simulink model "Sim_Forcing_003h_expe_infra_transz_lim"  (Simulink 7.4)
settings: Solver=FixedStepDiscrete  StartTime=0.0  StopTime=inf  FixedStep=0.004  RelTol=1e-3
undefined symbols (not defined in the file or in its folder): DiscIntNeverNeededParam
libraries: simulink x39, gt_rt_lib x22, xpcutilitieslib x4, xpclib x2, dspswit3 x1
(part 1 of 4)
CloseFcn:
  | rtwprivate ssgencode ModelCloseRequest test
settings Model: Creator=traenkle  LastModifiedBy=iMose1  SimulationMode=external  ExtModeTrigDuration=10000
settings OptimizationCC: LocalBlockOutputs=off  InitFltsAndDblsToZero=on
settings DebuggingCC: AlgebraicLoopMsg=error  ArtificialAlgebraicLoopMsg=error  SaveWithParameterizedLinksMsg=none  BlockPriorityViolationMsg=error  MinStepSizeMsg=error
settings HardwareCC: TargetEndianess=LittleEndian  TargetHWDeviceType=MATLAB Host
settings RTWCC: SystemTargetFile=gt_rt.tlc  TemplateMakefile=gt_rt.tmf  Description=GIGATRONIK Real-Time Target  ProcessScript=gt_rt_make_rtw_hook
settings STFCustomTargetCC: ModelReferenceCompliant=off  GeneratePreprocessorConditionals=Disable all  MatFileLogging=on  SystemTargetFile=gt_rt.tlc
settings GRTTargetCC: ModelReferenceCompliant=off  ParMdlRefBuildCompliant=off  CompOptLevelCompliant=off  ExtMode=on  ExtModeMexArgs='192.168.102.111'
settings CustomProperty: DataType=string  Value=gtrt

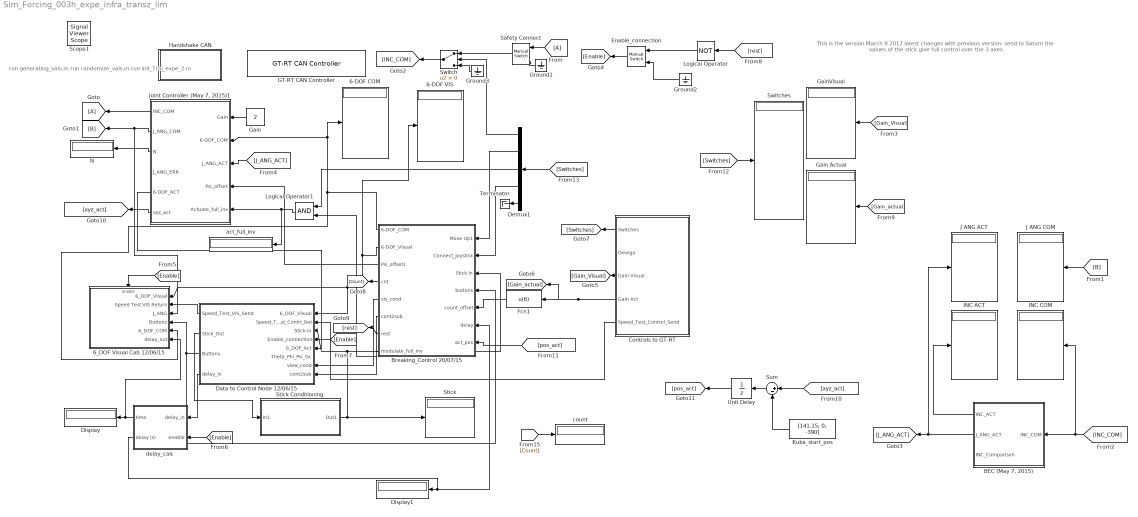
== system Sim_Forcing_003h_expe_infra_transz_lim ==
  note: This is the version
      | March 9 2017
      |
      | latest changes with previous version:
      | send to Saturn the values of the stick
      | give full control over the 3 axes
  note: run generating_vals.m
      | run randomize_vals.m
      | run init_Traj_expe_2.m
  6-DOF COM : Display
  6-DOF VIS : Display
  6_DOF Visual Cab 12/06/15 : Subsystem
  "BEC (May 7, 2015)" : Subsystem
  Breaking_Control 20/07/15 : Subsystem
  Controls to GT-RT : Subsystem
  Data to Control Node 12/06/15 : Subsystem
  Demux1 : Demux  Outputs=[1,1,1,3,4]
  Display : Display
  Display1 : Display
  Enable_connection : simulink/Signal Routing/Manual Switch  SystemSampleTime=-1  sw=1  action=0  varsize=off
  Fcn1 : Fcn  Expr=u(6)
  GT-RT CAN Controller : gt_rt_lib/GT-RT CAN Controller  uri='gt_rt_dev://localhost/dev/can0#0'  options='baudrate=500'
  Gain : Constant  Value=2  OutDataType=fixdt(1, 16)  OutScaling=2^0
  Gain Actual : Display
  GainVisual : Display
  Ground1 : Ground
  Ground2 : Ground
  Ground3 : Ground
  Handshake CAN : Subsystem
  INC ACT : Display
  INC COM : Display
  J ANG ACT : Display
  J ANG COM : Display
  "Joint Controller (May 7, 2015)1" : Subsystem
  Kuka_start_pos : Constant  Value=[141.15; 0; -390]  OutDataType=fixdt(1, 16)  OutScaling=2^0
  Logical Operator : Logic  Operator=NOT  AllPortsSameDT=off  OutDataTypeMode=boolean  LogicDataType=fixdt(0, 8)  OutDataTypeStr=boolean
  Logical Operator1 : Logic  AllPortsSameDT=off  OutDataTypeMode=boolean  LogicDataType=fixdt(0, 8)  OutDataTypeStr=boolean
  N : Display
  Safety Connect : simulink/Signal Routing/Manual Switch  SystemSampleTime=-1  sw=1  action=0  varsize=off
  Stick : Display
      settings: Decimation=40
  Stick Conditioning : Subsystem
  Sum : Sum  Inputs=|+-  OutDataType=fixdt(1, 16)  OutScaling=2^0
  Switch : Switch  Criteria=u2 > Threshold  OutDataType=fixdt(1, 16)  OutScaling=2^0
  Switches : Display
  Terminator : Terminator
  Unit Delay : UnitDelay  X0=[0 0 0]  SampleTime=-1
  act_full_inv : Display
  count : Display
      settings: Decimation=40
  delay_calc : Subsystem
  Scope1 : SignalViewerScope  IOType=viewer  ZoomMode=xonly  LegendLocations="524.3333           184           121      20.33333"  RefreshTime=0.035000
      settings: ShowLegends=on  TimeRange=10  YMin=2  YMax=3
  wires:
  Gain/1 -> "Joint Controller (May 7, 2015)1"/1(Gain)
  "Joint Controller (May 7, 2015)1"/1(INC_COM) -> [A]
  [A] -> Safety Connect/1
  "Joint Controller (May 7, 2015)1"/2(J_ANG_COM) -> [B], 6_DOF Visual Cab 12/06/15/3(J_ANG)
  "Joint Controller (May 7, 2015)1"/5(6-DOF_ACT) -> Data to Control Node 12/06/15/5(6_DOF_Act)
  [J_ANG_ACT] -> "Joint Controller (May 7, 2015)1"/3(J_ANG_ACT)
  "Joint Controller (May 7, 2015)1"/3(N) -> N/1
  Safety Connect/1 -> Switch/1
  Controls to GT-RT/3(Gain Visual) -> [Gain_Visual]
  Stick Conditioning/1(Out1) -> Stick/1, Breaking_Control 20/07/15/3(Stick In), Data to Control Node 12/06/15/3(Stick in)
  Data to Control Node 12/06/15/1(Speed_Test_VIS_Send) -> 6_DOF Visual Cab 12/06/15/2(Speed Test VIS Return)
  Controls to GT-RT/1(Switches) -> [Switches]
  Demux1/2 -> Breaking_Control 20/07/15/1(Move Up1)
  "BEC (May 7, 2015)"/2(J_ANG_ACT) -> [J_ANG_ACT], J ANG ACT/1
  Ground1/1 -> Safety Connect/2
  Ground3/1 -> Switch/3
  Demux1/1 -> Switch/2
  "BEC (May 7, 2015)"/1(INC_ACT) -> INC ACT/1
  [B] -> J ANG COM/1
  Switch/1 -> [INC_COM]
  [INC_COM] -> INC COM/1, "BEC (May 7, 2015)"/1(INC_COM)
  Breaking_Control 20/07/15/1(6-DOF_COM) -> 6-DOF COM/1, "Joint Controller (May 7, 2015)1"/2(6-DOF_COM), 6_DOF Visual Cab 12/06/15/5(6_DOF_COM)
  Demux1/4 -> Breaking_Control 20/07/15/2(Connect_Joystick)
  Demux1/5 -> Terminator/1
  Data to Control Node 12/06/15/3(Buttons) -> 6_DOF Visual Cab 12/06/15/4(Buttons), Breaking_Control 20/07/15/4(buttons)
  Breaking_Control 20/07/15/2(6-DOF_Visual) -> 6-DOF VIS/1, 6_DOF Visual Cab 12/06/15/1(6_DOF_Visual), Data to Control Node 12/06/15/1(6_DOF_Visual)
  Breaking_Control 20/07/15/3(Psi_offset1) -> "Joint Controller (May 7, 2015)1"/4(Psi_offset)
  Data to Control Node 12/06/15/4(delay_in) -> delay_calc/1(delay_in)
  delay_calc/1(time) -> Display/1, 6_DOF Visual Cab 12/06/15/6(delay_out)
  delay_calc/2(delay (s)) -> Display1/1, Breaking_Control 20/07/15/6(delay)
  Ground2/1 -> Enable_connection/2
  [Enable] -> 6_DOF Visual Cab 12/06/15/Enable
  [Enable] -> delay_calc/2(enable)
  [Enable] -> Data to Control Node 12/06/15/4(Enable_connection)
  [Gain_Visual] -> GainVisual/1
  [Gain_actual] -> Gain Actual/1
  Controls to GT-RT/4(Gain Act) -> [Gain_actual], Fcn1/1
  [Switches] -> Switches/1
  [Switches] -> Demux1/1
  Controls to GT-RT/5(Speed_Test_Control_Send) -> Data to Control Node 12/06/15/2(Speed_Test_Contrl_Ret)
  Enable_connection/1 -> [Enable]
  [Count] -> count/1
  Breaking_Control 20/07/15/4(cnt) -> [Count]
  Breaking_Control 20/07/15/5(vis_cond) -> Data to Control Node 12/06/15/7(view_cond)
  Breaking_Control 20/07/15/6(cont2sub) -> Data to Control Node 12/06/15/8(cont2sub)
  Breaking_Control 20/07/15/7(rest) -> [rest]
  [rest] -> Logical Operator/1
  Fcn1/1 -> Breaking_Control 20/07/15/5(count_offset)
  Unit Delay/1 -> [pos_act]
  [pos_act] -> Breaking_Control 20/07/15/7(act_pos)
  "Joint Controller (May 7, 2015)1"/6(xyz_act) -> [xyz_act]
  Sum/1 -> Unit Delay/1
  [xyz_act] -> Sum/1
  Kuka_start_pos/1 -> Sum/2
  Demux1/3 -> Logical Operator1/1
  Breaking_Control 20/07/15/8(modulate_full_inv) -> Logical Operator1/2
  Logical Operator1/1 -> "Joint Controller (May 7, 2015)1"/5(Actuate_full_inv), act_full_inv/1
  Logical Operator/1 -> Enable_connection/1
  Data to Control Node 12/06/15/2(Stick_Out) -> Stick Conditioning/1(In1)

== system Sim_Forcing_003h_expe_infra_transz_lim/6_DOF Visual Cab 12/06/15 ==
  note: send to visual node
  6_DOF_Visual : Inport
  Speed Test VIS Return : Inport  Port=2
  J_ANG : Inport  Port=3
  Buttons : Inport  Port=4
  6_DOF_COM : Inport  Port=5
  delay_out : Inport  Port=6
  Enable : EnablePort
  "Byte Packing " : xpcutilitieslib/Byte Packing   MaskPackedDataType=uint8  MaskUnpackedDataTypes={'single','single','single'}  MaskAlignment=1
  Constant2 : Constant  Value=9200  OutDataTypeMode=uint16  OutDataType=fixdt(1, 16)  OutScaling=2^0  OutDataTypeStr=uint16
  Constant3 : Constant  Value=32  OutDataTypeMode=uint32  OutDataType=fixdt(1, 16)  OutScaling=2^0  OutDataTypeStr=uint32
  Data Type Conversion : DataTypeConversion  OutDataTypeMode=single  OutDataType=fixdt(1, 16)  OutScaling=2^0  OutDataTypeStr=single
  Data Type Conversion1 : DataTypeConversion  OutDataTypeMode=single  OutDataType=fixdt(1, 16)  OutScaling=2^0  OutDataTypeStr=single
  Data Type Conversion6 : DataTypeConversion  OutDataTypeMode=single  OutDataType=fixdt(1, 16)  OutScaling=2^0  OutDataTypeStr=single
  GT-RT UDP  Write : gt_rt_lib/GT-RT UDP  Controller  uri='gtp://localhost/udp?port=9200'
  GT-RT UDP TX : gt_rt_lib/GT-RT UDP TX  uri='gtp://localhost/udp?port=9200'  hostname='192.168.102.13'
  Write Error : Display
  wires:
  Constant2/1 -> GT-RT UDP TX/2
  GT-RT UDP TX/1 -> Write Error/1
  Constant3/1 -> GT-RT UDP TX/4
  "Byte Packing "/1 -> GT-RT UDP TX/3
  Speed Test VIS Return/1 -> Data Type Conversion1/1
  6_DOF_Visual/1 -> Data Type Conversion/1
  Data Type Conversion1/1 -> "Byte Packing "/2
  Data Type Conversion/1 -> "Byte Packing "/1
  delay_out/1 -> Data Type Conversion6/1
  Data Type Conversion6/1 -> "Byte Packing "/3

== system Sim_Forcing_003h_expe_infra_transz_lim/BEC (May 7, 2015) ==
  INC_COM : Inport
  CAN Receive : Subsystem
  CAN Send : Subsystem
  Demux : Demux  Outputs=6
  Demux1 : Demux  Outputs=6
  Mux : Mux  Inputs=6
  Mux2 : Mux  Inputs=6
  Software limit switches : Subsystem
  Sum1 : Sum  Inputs=-+|  OutDataType=fixdt(1, 16)  OutScaling=2^0
  velocity and acceleration limitation : Subsystem
  INC_ACT : Outport
  J_ANG_ACT : Outport  Port=2
  INC_Comparison : Outport  Port=3
  wires:
  CAN Receive/7(New Data Flag (93)) -> CAN Send/1(New data flag (93))
  velocity and acceleration limitation/3(A3) -> Mux2/3
  velocity and acceleration limitation/6(A6) -> Mux2/6
  velocity and acceleration limitation/1(A1) -> Mux2/1
  velocity and acceleration limitation/2(A2) -> Mux2/2
  velocity and acceleration limitation/4(A4) -> Mux2/4
  velocity and acceleration limitation/5(A5) -> Mux2/5
  Software limit switches/1(Out1) -> velocity and acceleration limitation/1(In1)
  Software limit switches/2(Out2) -> velocity and acceleration limitation/2(In2)
  Software limit switches/3(Out3) -> velocity and acceleration limitation/3(In3)
  Software limit switches/4(Out4) -> velocity and acceleration limitation/4(In4)
  Software limit switches/5(Out5) -> velocity and acceleration limitation/5(In5)
  Software limit switches/6(Out6) -> velocity and acceleration limitation/6(In6)
  CAN Receive/1(Act_Axis1 [deg]) -> Mux/1
  CAN Receive/2(Act_Axis2  [deg]) -> Mux/2
  CAN Receive/3(Act_Axis3  [deg]) -> Mux/3
  CAN Receive/4(Act_Axis4 [deg]) -> Mux/4
  CAN Receive/5(Act_Axis5 [deg]) -> Mux/5
  CAN Receive/6(Act_Axis6 [deg]) -> Mux/6
  Demux/1 -> Software limit switches/1(In1)
  Demux/2 -> Software limit switches/2(In2)
  Demux/3 -> Software limit switches/3(In3)
  Demux/4 -> Software limit switches/4(In4)
  Demux/5 -> Software limit switches/5(In5)
  Demux/6 -> Software limit switches/6(In6)
  Mux/1 -> J_ANG_ACT/1, Software limit switches/7(act)
  INC_COM/1 -> Demux/1, Sum1/2
  Mux2/1 -> INC_ACT/1, Sum1/1, Demux1/1
  Sum1/1 -> INC_Comparison/1
  Demux1/1 -> CAN Send/2(A1 [deg/4ms])
  Demux1/2 -> CAN Send/3(A2 [deg/4ms])
  Demux1/3 -> CAN Send/4(A3 [deg/4ms])
  Demux1/4 -> CAN Send/5(A4 [deg/4ms])
  Demux1/5 -> CAN Send/6(A5 [deg/4ms])
  Demux1/6 -> CAN Send/7(A6 [deg/4ms])

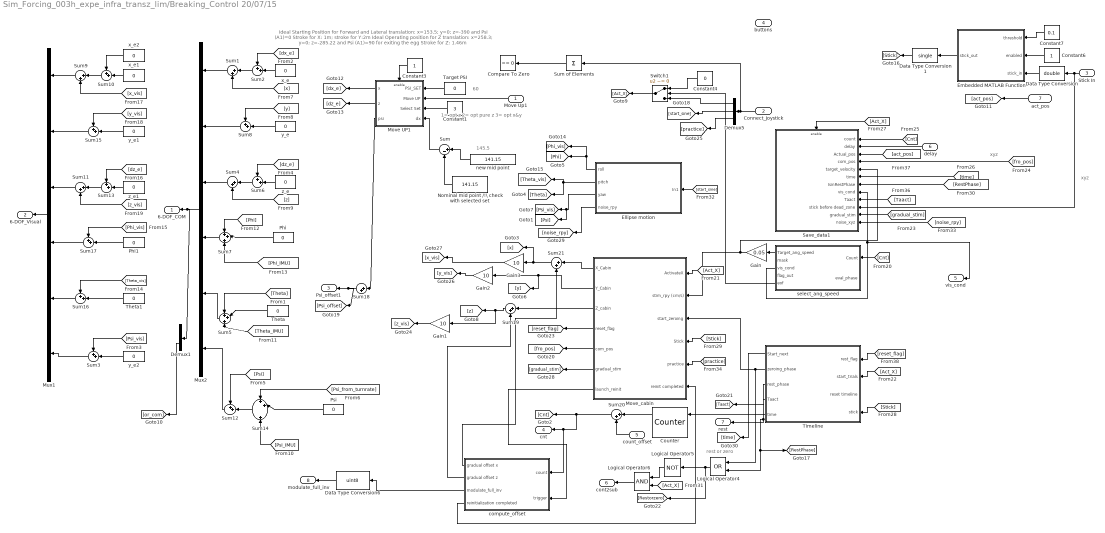
== system Sim_Forcing_003h_expe_infra_transz_lim/Breaking_Control 20/07/15 ==
  note: Ideal Starting Position for Forward and Lateral translation:
      | x=153.5; y=0; z=-390 and Psi (A1)=0
      | Stroke for X: 1m; stroke for Y:2m
      | Ideal Operating position for Z translation:
      | x=258.3; y=0; z=-285.22 and Psi (A1)=90 for exiting the egg
      | Stroke for Z: 1.46m
  note: 1= opt z
      | 2= opt pure z
      | 3= opt x&y
  note: 60
  note: 145.5
  note: rest or zero
  note: xyz
  note: xyz
  Move Up1 : Inport  OutDataType=fixdt(1, 16)  OutScaling=2^0
  Connect_Joystick : Inport  Port=2  OutDataType=fixdt(1, 16)  OutScaling=2^0
  Stick In : Inport  Port=3  OutDataType=fixdt(1, 16)  OutScaling=2^0
  buttons : Inport  Port=4  OutDataType=fixdt(1, 16)  OutScaling=2^0
  count_offset : Inport  Port=5  OutDataType=fixdt(1, 16)  OutScaling=2^0
  delay : Inport  Port=6  OutDataType=fixdt(1, 16)  OutScaling=2^0
  act_pos : Inport  Port=7  OutDataType=fixdt(1, 16)  OutScaling=2^0
  Compare To Zero : simulink/Logic and Bit Operations/Compare To Zero  SystemSampleTime=-1  relop===  LogicOutDataTypeMode=uint8
  Constant1 : Constant  Value=3  OutDataType=fixdt(1, 16)  OutScaling=2^0
  Constant3 : Constant  OutDataType=fixdt(1, 16)  OutScaling=2^0
  Constant4 : Constant  Value=0  OutDataType=fixdt(1, 16)  OutScaling=2^0
  Constant6 : Constant  OutDataType=fixdt(1, 16)  OutScaling=2^0
  Constant7 : Constant  Value=0.1  OutDataType=fixdt(1, 16)  OutScaling=2^0
  Counter : dspswit3/Counter  Direction=Up  CountEvent=Rising edge  CounterSize=User defined  MaxCount=200  InitialCount=1  Output=Count and Hit  HitValue=32  ResetInput=on  SamplesPerFrame=1  Ts=1  CntDtype=double  HitDtype=Logical
  Data Type Conversion : DataTypeConversion  OutDataTypeMode=double  OutDataType=fixdt(1, 16)  OutScaling=2^0  OutDataTypeStr=double
  Data Type Conversion1 : DataTypeConversion  OutDataTypeMode=single  OutDataType=fixdt(1, 16)  OutScaling=2^0  OutDataTypeStr=single
  Data Type Conversion6 : DataTypeConversion  OutDataTypeMode=uint8  OutDataType=fixdt(1, 16)  OutScaling=2^0  OutDataTypeStr=uint8
  Demux1 : Demux  Outputs=[3 3]
  Demux5 : Demux  Outputs=3
  Ellipse motion : Subsystem
  Embedded MATLAB Function : Stateflow chart
  Gain : Gain  Gain=0.05  ParameterDataType=fixdt(1, 16)  ParameterScaling=2^0  OutDataType=fixdt(1, 16)  OutScaling=2^0
  Gain1 : Gain  Gain=10  ParameterDataType=fixdt(1, 16)  ParameterScaling=2^0  OutDataType=fixdt(1, 16)  OutScaling=2^0
  Gain2 : Gain  Gain=10  ParameterDataType=fixdt(1, 16)  ParameterScaling=2^0  OutDataType=fixdt(1, 16)  OutScaling=2^0
  Gain3 : Gain  Gain=10  ParameterDataType=fixdt(1, 16)  ParameterScaling=2^0  OutDataType=fixdt(1, 16)  OutScaling=2^0
  Logical Operator4 : Logic  Operator=OR  AllPortsSameDT=off  OutDataTypeMode=boolean  LogicDataType=fixdt(0, 8)  OutDataTypeStr=boolean
  Logical Operator5 : Logic  Operator=NOT  AllPortsSameDT=off  OutDataTypeMode=boolean  LogicDataType=fixdt(0, 8)  OutDataTypeStr=boolean
  Logical Operator6 : Logic  AllPortsSameDT=off  OutDataTypeMode=boolean  LogicDataType=fixdt(0, 8)  OutDataTypeStr=boolean
  Move UP1 : Subsystem
  Move_cabin : Subsystem
  Mux1 : Mux  Inputs=6
  Mux2 : Mux  Inputs=6
  Nominal mid point /!\ check with selected set : Constant  Value=141.15  OutDataType=fixdt(1, 16)  OutScaling=2^0
  Phi : Constant  Value=0  OutDataType=fixdt(1, 16)  OutScaling=2^0
  Phi1 : Constant  Value=0  OutDataType=fixdt(1, 16)  OutScaling=2^0
  Psi : Constant  Value=0  OutDataType=fixdt(1, 16)  OutScaling=2^0
  Save_data1 : Subsystem
  Sum : Sum  Inputs=|+-  OutDataType=fixdt(1, 16)  OutScaling=2^0
  Sum of Elements : Sum  Inputs=+  OutDataType=fixdt(1, 16)  OutScaling=2^-10
  Sum{1,4,9,11,18..21} (8 alike) : Sum  Inputs=|++  OutDataType=fixdt(1, 16)  OutScaling=2^0
  Sum{2..3,6,8,10,12..13,15..17} (10 alike) : Sum  Inputs=++|  OutDataType=fixdt(1, 16)  OutScaling=2^0
  Sum14 : Sum  Inputs=++|+  OutDataType=fixdt(1, 16)  OutScaling=2^0
  Sum5 : Sum  Inputs=++|+  OutDataType=fixdt(1, 16)  OutScaling=2^0
  Sum7 : Sum  Inputs=++|+  OutDataType=fixdt(1, 16)  OutScaling=2^0
  Switch1 : Switch  Criteria=u2 ~= 0  OutDataType=fixdt(1, 16)  OutScaling=2^0
  Target PSI : Constant  Value=0  OutDataType=fixdt(1, 16)  OutScaling=2^0
  Theta : Constant  Value=0  OutDataType=fixdt(1, 16)  OutScaling=2^0
  Theta1 : Constant  Value=0  OutDataType=fixdt(1, 16)  OutScaling=2^0
  Timeline : Subsystem
  compute_offset : Subsystem
  new mid point : Constant  Value=141.15  OutDataType=fixdt(1, 16)  OutScaling=2^0
  select_ang_speed : Subsystem
  x_e : Constant  Value=0  OutDataType=fixdt(1, 16)  OutScaling=2^0
  x_e1 : Constant  Value=0  OutDataType=fixdt(1, 16)  OutScaling=2^0
  x_e2 : Constant  Value=0  OutDataType=fixdt(1, 16)  OutScaling=2^0
  y_e : Constant  Value=0  OutDataType=fixdt(1, 16)  OutScaling=2^0
  y_e1 : Constant  Value=0  OutDataType=fixdt(1, 16)  OutScaling=2^0
  y_e2 : Constant  Value=0  OutDataType=fixdt(1, 16)  OutScaling=2^0
  z_e : Constant  Value=0  OutDataType=fixdt(1, 16)  OutScaling=2^0
  z_e1 : Constant  Value=0  OutDataType=fixdt(1, 16)  OutScaling=2^0
  6-DOF_COM : Outport
  6-DOF_Visual : Outport  Port=2
  Psi_offset1 : Outport  Port=3
  cnt : Outport  Port=4
  vis_cond : Outport  Port=5
  cont2sub : Outport  Port=6
  rest : Outport  Port=7
  modulate_full_inv : Outport  Port=8
  wires:
  Connect_Joystick/1 -> Sum of Elements/1, Demux5/1
  Move Up1/1 -> Move UP1/2(Move UP)
  Constant1/1 -> Move UP1/3(Select Set)
  Sum of Elements/1 -> Compare To Zero/1
  Move UP1/1(x) -> [dx_e]
  Mux2/1 -> 6-DOF_COM/1, Demux1/1
  Sum1/1 -> Mux2/1
  Sum5/1 -> Mux2/5
  [Theta] -> Sum5/1
  Sum4/1 -> Mux2/3
  [Phi] -> Sum7/1
  Sum7/1 -> Mux2/4
  y_e/1 -> Sum8/2
  Sum8/1 -> Mux2/2
  [dx_e] -> Sum2/1
  x_e/1 -> Sum2/2
  Sum2/1 -> Sum1/1
  z_e/1 -> Sum6/2
  [dz_e] -> Sum6/1
  Sum6/1 -> Sum4/1
  Sum13/1 -> Sum11/1
  z_e1/1 -> Sum13/2
  Sum10/1 -> Sum9/1
  x_e1/1 -> Sum10/2
  x_e2/1 -> Sum10/1
  Sum15/1 -> Mux1/2
  y_e1/1 -> Sum15/2
  Sum11/1 -> Mux1/3
  Sum9/1 -> Mux1/1
  Mux1/1 -> 6-DOF_Visual/1
  Theta/1 -> Sum5/2
  Phi/1 -> Sum7/2
  Sum3/1 -> Mux1/6
  [Psi_vis] -> Sum3/1
  y_e2/1 -> Sum3/2
  Sum12/1 -> Mux2/6
  [Psi] -> Sum12/1
  Nominal mid point /!\ check with selected set/1 -> Sum/2
  new mid point/1 -> Sum/1
  Move UP1/2(z) -> [dz_e]
  Target PSI/1 -> Move UP1/1(PSI_SET)
  Sum/1 -> Move UP1/4(dx)
  Sum14/1 -> Sum12/2
  [Psi_from_turnrate] -> Sum14/1
  Psi/1 -> Sum14/2
  [Psi_IMU] -> Sum14/3
  [Theta_IMU] -> Sum5/3
  [Phi_IMU] -> Sum7/3
  Theta1/1 -> Sum16/2
  Sum16/1 -> Mux1/5
  Sum17/1 -> Mux1/4
  Phi1/1 -> Sum17/2
  [Theta_vis] -> Sum16/1
  [Phi_vis] -> Sum17/1
  Timeline/1(Start_next) -> Counter/1
  [Cnt] -> select_ang_speed/1(Count)
  Timeline/2(zeroing_phase) -> Move_cabin/3(start_zeroing), Logical Operator4/1
  Timeline/3(rest_phase) -> Logical Operator4/2, [RestPhase], rest/1
  delay/1 -> Save_data1/2(delay)
  [Act_X] -> Move_cabin/1(ActivateX)
  [Act_X] -> Timeline/2(start_trials)
  Demux1/2 -> [or_com]
  [Cnt] -> Save_data1/1(count)
  [time] -> Save_data1/6(time)
  Logical Operator4/1 -> [Restorzero], Logical Operator5/1
  [dz_e] -> Sum13/1
  Constant3/1 -> Move UP1/Enable
  [x_vis] -> Sum9/2
  [y_vis] -> Sum15/1
  [z_vis] -> Sum11/2
  [x] -> Sum1/2
  [y] -> Sum8/1
  [z] -> Sum4/2
  [Stick] -> Timeline/4(stick)
  [RestPhase] -> Save_data1/7(IsinRestPhase)
  [Act_X] -> Save_data1/Enable
  select_ang_speed/3(vis_cond) -> Save_data1/8(vis_cond), vis_cond/1
  select_ang_speed/1(Target_ang_speed) -> Gain/1
  Sum18/1 -> Psi_offset1/1, [Psi_offset]
  Move UP1/3(psi) -> Sum18/1
  Gain/1 -> Save_data1/5(target_velocity), Move_cabin/2(stim_rpy (cm/s))
  [Act_X] -> Logical Operator6/2
  Logical Operator6/1 -> cont2sub/1
  Logical Operator5/1 -> Logical Operator6/1
  [fro_pos] -> Save_data1/4(com_pos)
  Counter/1 -> Sum20/1
  count_offset/1 -> Sum20/2
  Sum20/1 -> [Cnt], cnt/1, compute_offset/1(count)
  Timeline/4(Taact) -> [Taact]
  [Taact] -> Save_data1/9(Taact)
  [act_pos] -> Save_data1/3(Actual_pos)
  Switch1/1 -> [Act_X]
  Constant4/1 -> Switch1/1
  Demux5/1 -> Switch1/3
  select_ang_speed/5(eof) -> Switch1/2
  Embedded MATLAB Function/1(stick_out) -> Data Type Conversion1/1
  Stick In/1 -> Data Type Conversion/1, Save_data1/10(stick before dead_zone)
  Constant6/1 -> Embedded MATLAB Function/2(enabled)
  Constant7/1 -> Embedded MATLAB Function/1(threshold)
  Demux5/3 -> [practice]
  Data Type Conversion/1 -> Embedded MATLAB Function/3(stick_in)
  Data Type Conversion1/1 -> [Stick]
  [Stick] -> Move_cabin/4(Stick)
  Move_cabin/4(reset_flag) -> [reset_flag]
  [reset_flag] -> Timeline/1(rest_flag)
  Move_cabin/5(com_pos) -> [fro_pos]
  act_pos/1 -> [act_pos]
  [practice] -> Move_cabin/5(practice)
  Demux5/2 -> [start_sine]
  [start_sine] -> Ellipse motion/1(In1)
  Move_cabin/6(gradual_stim) -> [gradual_stim]
  [gradual_stim] -> Save_data1/11(gradual_stim)
  [noise_rpy] -> Save_data1/12(noise_xyz)
  Timeline/5(time) -> [time]
  Move_cabin/2(Y_Cabin) -> [y], Gain2/1
  Ellipse motion/4(noise_rpy) -> [noise_rpy]
  Ellipse motion/2(pitch) -> [Theta], [Theta_vis]
  Ellipse motion/1(roll) -> [Phi], [Phi_vis]
  Ellipse motion/3(yaw) -> [Psi_vis], [Psi]
  Gain1/1 -> [z_vis]
  Gain2/1 -> [y_vis]
  Gain3/1 -> [x_vis]
  compute_offset/4(reinitialization completed) -> Move_cabin/6(reinit completed)
  Move_cabin/7(launch_reinit) -> compute_offset/2(trigger)
  Sum19/1 -> [z], Gain1/1
  Move_cabin/3(Z_cabin) -> Sum19/1
  compute_offset/2(gradual offset z) -> Sum19/2
  Sum21/1 -> Gain3/1, [x]
  Move_cabin/1(X_Cabin) -> Sum21/1
  compute_offset/1(gradual offset x) -> Sum21/2
  compute_offset/3(modulate_full_inv) -> Data Type Conversion6/1
  Data Type Conversion6/1 -> modulate_full_inv/1

== system Sim_Forcing_003h_expe_infra_transz_lim/Controls to GT-RT ==
  Display2 : Display
  Display4 : Display
  Display5 : Display
  Error : Display
  GT-RT UDP  Read : gt_rt_lib/GT-RT UDP  Controller  uri='gtp://localhost/udp?port=9500'
  GT-RT UDP RX : gt_rt_lib/GT-RT UDP RX  uri='gtp://localhost/udp?port=9500'  receive_buffer_size=66  timeout=0  sample_time=0.004
  Terminator : Terminator
  Unpack : xpclib/UDP/Unpack  dimensions={10,1,6,6,1}  datatypes={'uint8','single','single','single','single'}  byteAlign=1
  Switches : Outport  OutDataType=fixdt(1, 16)  OutScaling=2^0
  Omega : Outport  Port=2  OutDataType=fixdt(1, 16)  OutScaling=2^0
  Gain Visual : Outport  Port=3  OutDataType=fixdt(1, 16)  OutScaling=2^0
  Gain Act : Outport  Port=4  OutDataType=fixdt(1, 16)  OutScaling=2^0
  Speed_Test_Control_Send : Outport  Port=5  OutDataType=fixdt(1, 16)  OutScaling=2^0
  wires:
  GT-RT UDP RX/2 -> Display2/1
  GT-RT UDP RX/6 -> Error/1
  GT-RT UDP RX/5 -> Display4/1
  GT-RT UDP RX/4 -> Display5/1
  GT-RT UDP RX/1 -> Unpack/1
  GT-RT UDP RX/3 -> Terminator/1
  Unpack/1 -> Switches/1
  Unpack/2 -> Omega/1
  Unpack/3 -> Gain Act/1
  Unpack/4 -> Gain Visual/1
  Unpack/5 -> Speed_Test_Control_Send/1

== system Sim_Forcing_003h_expe_infra_transz_lim/Data to Control Node 12/06/15 ==
  6_DOF_Visual : Inport
  Speed_Test_Contrl_Ret : Inport  Port=2
  Stick in : Inport  Port=3
  Enable_connection : Inport  Port=4
  6_DOF_Act : Inport  Port=5
  Theta_Phi_Psi_Oc : Inport  Port=6
  view_cond : Inport  Port=7
  cont2sub : Inport  Port=8
  6_DOF Control : Subsystem
  "Interaction device from VIS (Stick) " : Subsystem
  Speed_Test_VIS_Send : Outport  OutDataType=fixdt(1, 16)  OutScaling=2^0
  Stick_Out : Outport  Port=2  OutDataType=fixdt(1, 16)  OutScaling=2^0
  Buttons : Outport  Port=3  OutDataType=fixdt(1, 16)  OutScaling=2^0
  delay_in : Outport  Port=4  OutDataType=fixdt(1, 16)  OutScaling=2^0
  wires:
  6_DOF_Visual/1 -> 6_DOF Control/1(6_DOF_Visual)
  "Interaction device from VIS (Stick) "/1(Stick Out) -> Stick_Out/1
  "Interaction device from VIS (Stick) "/2(Buttons) -> 6_DOF Control/3(Buttons), Buttons/1
  Speed_Test_Contrl_Ret/1 -> 6_DOF Control/4(Speed Test Control Return)
  "Interaction device from VIS (Stick) "/3(Speed_Test_VIS_Send) -> Speed_Test_VIS_Send/1
  Stick in/1 -> 6_DOF Control/2(Stick In)
  Enable_connection/1 -> 6_DOF Control/Enable
  6_DOF_Act/1 -> 6_DOF Control/5(6_DOF_Act)
  Theta_Phi_Psi_Oc/1 -> 6_DOF Control/6(Theta_Phi_Psi_Oc)
  "Interaction device from VIS (Stick) "/4(for_delay_calc) -> delay_in/1
  view_cond/1 -> 6_DOF Control/7(view_cond)
  cont2sub/1 -> 6_DOF Control/8(cont2sub)

== system Sim_Forcing_003h_expe_infra_transz_lim/Handshake CAN ==
  GT-RT CAN RX2 : gt_rt_lib/GT-RT CAN RX  uri='gt_rt_dev://localhost/dev/can0#0'  receive_all_can_ids=off  can_id=hex2dec('90')  sample_time=-1
  If : If  IfExpression=u1 ~= 0  ShowElse=off
  If Action Subsystem : Subsystem  TreatAsAtomicUnit=on
  If Action Subsystem1 : Subsystem  TreatAsAtomicUnit=on
  Terminator{1..5} (5 alike) : Terminator
  wires:
  GT-RT CAN RX2/5 -> If/1
  If/1 -> If Action Subsystem1/Action
  GT-RT CAN RX2/1 -> Terminator1/1
  GT-RT CAN RX2/2 -> Terminator2/1
  GT-RT CAN RX2/3 -> Terminator3/1
  GT-RT CAN RX2/4 -> Terminator4/1
  GT-RT CAN RX2/6 -> Terminator5/1

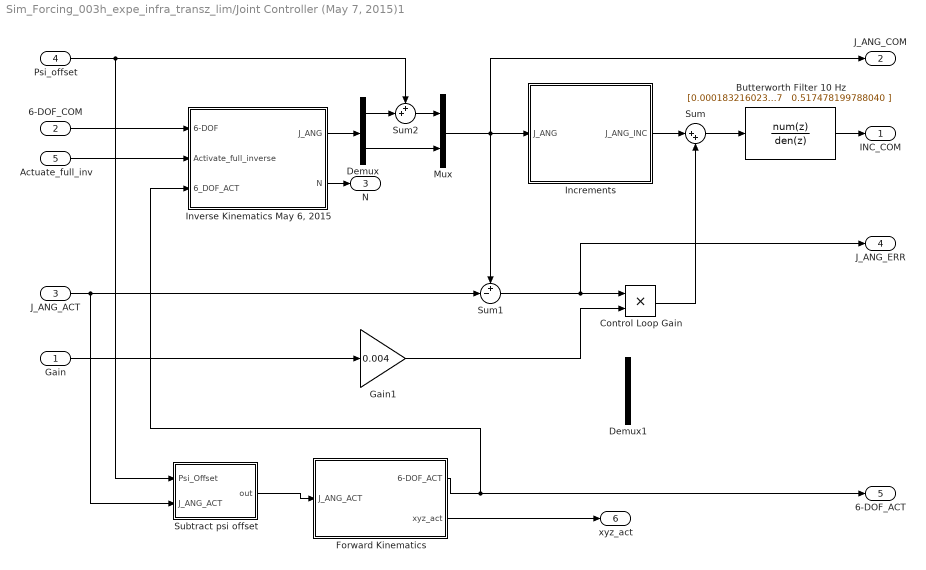
== system Sim_Forcing_003h_expe_infra_transz_lim/Joint Controller (May 7, 2015)1 ==
  Gain : Inport  OutDataType=fixdt(1, 16)  OutScaling=2^0
  6-DOF_COM : Inport  Port=2  OutDataType=fixdt(1, 16)  OutScaling=2^0
  J_ANG_ACT : Inport  Port=3  OutDataType=fixdt(1, 16)  OutScaling=2^0
  Psi_offset : Inport  Port=4  OutDataType=fixdt(1, 16)  OutScaling=2^0
  Actuate_full_inv : Inport  Port=5  OutDataType=fixdt(1, 16)  OutScaling=2^0
  Butterworth Filter 10 Hz : DiscreteTransferFcn  Numerator="[0.000183216023369   0.000732864093478   0.001099296140221   0.000732864093475   0.000183216023371]"  Denominator=|  SampleTime=0.004
      | [1.000000000000000  -3.344067837711873   4.238863950884063  -2.409342856586317   0.517478199788040
      | ]
  Control Loop Gain : Product  OutDataType=fixdt(1, 16)  OutScaling=2^0  RndMeth=Zero
  Demux : Demux  Outputs=[1,5]
  Demux1 : Demux  Outputs=[3,3]
  Forward Kinematics : Subsystem
  Gain1 : Gain  Gain=0.004  ParameterDataType=fixdt(1, 16)  ParameterScaling=2^0  OutDataType=fixdt(1, 16)  OutScaling=2^0
  Increments : Subsystem
  "Inverse Kinematics May 6, 2015" : Subsystem
  Mux : Mux  Inputs=[1,5]
  Subtract psi offset : Subsystem
  Sum : Sum  Inputs=|++  OutDataType=fixdt(1, 16)  OutScaling=2^0
  Sum1 : Sum  Inputs=+-|  OutDataType=fixdt(1, 16)  OutScaling=2^0
  Sum2 : Sum  Inputs=++|  OutDataType=fixdt(1, 16)  OutScaling=2^0
  INC_COM : Outport  OutDataType=fixdt(1, 16)  OutScaling=2^0
  J_ANG_COM : Outport  Port=2  OutDataType=fixdt(1, 16)  OutScaling=2^0
  N : Outport  Port=3  OutDataType=fixdt(1, 16)  OutScaling=2^0
  J_ANG_ERR : Outport  Port=4  OutDataType=fixdt(1, 16)  OutScaling=2^0
  6-DOF_ACT : Outport  Port=5  OutDataType=fixdt(1, 16)  OutScaling=2^0
  xyz_act : Outport  Port=6  OutDataType=fixdt(1, 16)  OutScaling=2^0
  wires:
  6-DOF_COM/1 -> "Inverse Kinematics May 6, 2015"/1(6-DOF)
  "Inverse Kinematics May 6, 2015"/1(J_ANG) -> Demux/1
  Increments/1(J_ANG_INC) -> Sum/1
  Sum1/1 -> J_ANG_ERR/1, Control Loop Gain/1
  J_ANG_ACT/1 -> Sum1/2, Subtract psi offset/2(J_ANG_ACT)
  Control Loop Gain/1 -> Sum/2
  Gain/1 -> Gain1/1
  Gain1/1 -> Control Loop Gain/2
  "Inverse Kinematics May 6, 2015"/2(N) -> N/1
  Sum/1 -> Butterworth Filter 10 Hz/1
  Butterworth Filter 10 Hz/1 -> INC_COM/1
  Forward Kinematics/1(6-DOF_ACT) -> 6-DOF_ACT/1, "Inverse Kinematics May 6, 2015"/3(6_DOF_ACT)
  Psi_offset/1 -> Subtract psi offset/1(Psi_Offset), Sum2/1
  Demux/1 -> Sum2/2
  Demux/2 -> Mux/2
  Subtract psi offset/1(out) -> Forward Kinematics/1(J_ANG_ACT)
  Actuate_full_inv/1 -> "Inverse Kinematics May 6, 2015"/2(Activate_full_inverse)
  Sum2/1 -> Mux/1
  Mux/1 -> Increments/1(J_ANG), Sum1/1, J_ANG_COM/1
  Forward Kinematics/2(xyz_act) -> xyz_act/1

== system Sim_Forcing_003h_expe_infra_transz_lim/Stick Conditioning ==
  note: roll
  note: pitch
  note: yaw
  In1 : Inport
  Butterworth Filter 10 Hz : DiscreteTransferFcn  Numerator="[0.000183216023369   0.000732864093478   0.001099296140221   0.000732864093475   0.000183216023371]"  Denominator=|  SampleTime=0.004
      | [1.000000000000000  -3.344067837711873   4.238863950884063  -2.409342856586317   0.517478199788040
      | ]
  Demux : Demux  Outputs=3
  Gain1 : Gain  Gain=1/32768.  ParameterDataType=fixdt(1, 16)  ParameterScaling=2^0  OutDataType=fixdt(1, 16)  OutScaling=2^0
  Gain2 : Gain  Gain=-1  ParameterDataType=fixdt(1, 16)  ParameterScaling=2^0  OutDataType=fixdt(1, 16)  OutScaling=2^0
  Gain3 : Gain  Gain=-1  ParameterDataType=fixdt(1, 16)  ParameterScaling=2^0  OutDataType=fixdt(1, 16)  OutScaling=2^0
  Mux : Mux  Inputs=3
  Reset roll joystick : Constant  Value=0  VectorParams1D=off  OutDataTypeMode=double  OutDataType=fixdt(1, 16)  OutScaling=2^0  OutDataTypeStr=double
  Reset yaw joystick : Constant  Value=0  VectorParams1D=off  OutDataTypeMode=double  OutDataType=fixdt(1, 16)  OutScaling=2^0  OutDataTypeStr=double
  Sum18 : Sum  Inputs=|++  OutDataType=fixdt(1, 16)  OutScaling=2^0  SampleTime=-1.0  OutDataTypeStr=Inherit: Same as first input
  Sum2 : Sum  Inputs=|++  OutDataType=fixdt(1, 16)  OutScaling=2^0  SampleTime=-1.0  OutDataTypeStr=Inherit: Same as first input
  Out1 : Outport
  wires:
  Gain1/1 -> Out1/1
  In1/1 -> Butterworth Filter 10 Hz/1
  Butterworth Filter 10 Hz/1 -> Demux/1
  Mux/1 -> Gain1/1
  Demux/2 -> Gain2/1
  Demux/1 -> Mux/2
  Demux/3 -> Gain3/1
  Reset yaw joystick/1 -> Sum18/2
  Reset roll joystick/1 -> Sum2/2
  Gain3/1 -> Mux/3
  Gain2/1 -> Mux/1

== system Sim_Forcing_003h_expe_infra_transz_lim/delay_calc ==
  delay_in : Inport
  enable : Inport  Port=2
  Constant : Constant  Value=0.01  OutDataType=fixdt(1, 16)  OutScaling=2^0
  Discrete-Time Integrator : DiscreteIntegrator  gainval=1  ExternalReset=either  SampleTime=0.004  OutDataType=fixdt(1, 16)  OutScaling=2^0  ICPrevOutput=DiscIntNeverNeededParam  ICPrevScaledInput=DiscIntNeverNeededParam
  Divide : Product  Inputs=*/  OutDataType=fixdt(1, 16)  OutScaling=2^-10
  Sum : Sum  Inputs=+|-  OutDataType=fixdt(1, 16)  OutScaling=2^0
  time : Outport
  delay (s) : Outport  Port=2
  wires:
  Discrete-Time Integrator/1 -> time/1, Sum/1
  Constant/1 -> Discrete-Time Integrator/1, Divide/2
  delay_in/1 -> Sum/2
  Sum/1 -> Divide/1
  Divide/1 -> delay (s)/1
  enable/1 -> Discrete-Time Integrator/2

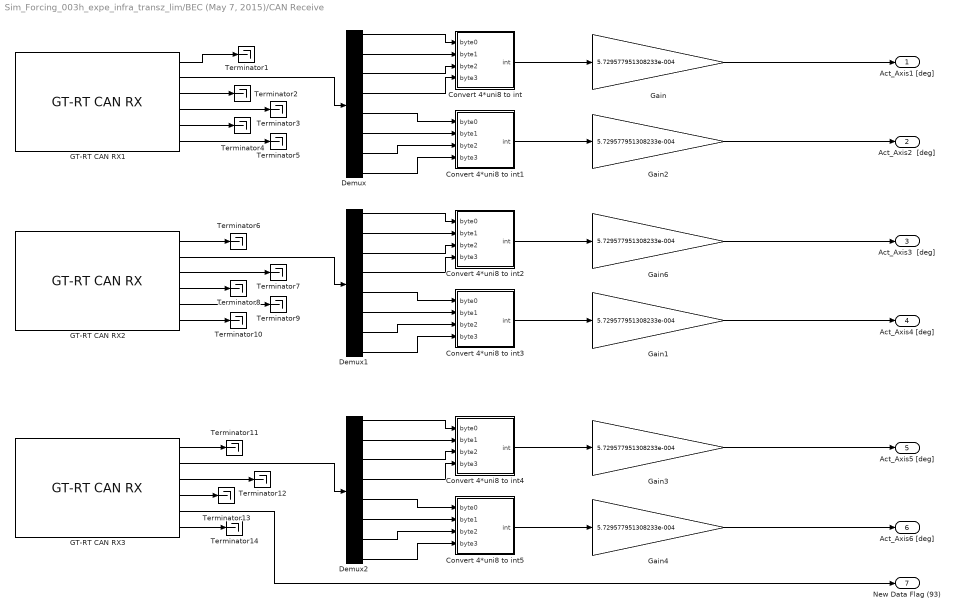
== system Sim_Forcing_003h_expe_infra_transz_lim/BEC (May 7, 2015)/CAN Receive ==
  Convert 4*uni8 to int : Subsystem
  Convert 4*uni8 to int1 : Subsystem
  Convert 4*uni8 to int2 : Subsystem
  Convert 4*uni8 to int3 : Subsystem
  Convert 4*uni8 to int4 : Subsystem
  Convert 4*uni8 to int5 : Subsystem
  Demux : Demux  Outputs=8
  Demux1 : Demux  Outputs=8
  Demux2 : Demux  Outputs=8
  GT-RT CAN RX1 : gt_rt_lib/GT-RT CAN RX  uri='gt_rt_dev://localhost/dev/can0#0'  receive_all_can_ids=off  can_id=hex2dec('91')  sample_time=-1
  GT-RT CAN RX2 : gt_rt_lib/GT-RT CAN RX  uri='gt_rt_dev://localhost/dev/can0#0'  receive_all_can_ids=off  can_id=hex2dec('92')  sample_time=-1
  GT-RT CAN RX3 : gt_rt_lib/GT-RT CAN RX  uri='gt_rt_dev://localhost/dev/can0#0'  receive_all_can_ids=off  can_id=hex2dec('93')  sample_time=-1
  Gain{,1..4,6} (6 alike) : Gain  Gain=5.729577951308233e-004  ParameterDataType=fixdt(1, 16)  ParameterScaling=2^0  OutDataType=fixdt(1, 16)  OutScaling=2^0
  Terminator{1..14} (14 alike) : Terminator
  Act_Axis1 [deg] : Outport
  Act_Axis2  [deg] : Outport  Port=2
  Act_Axis3  [deg] : Outport  Port=3
  Act_Axis4 [deg] : Outport  Port=4
  Act_Axis5 [deg] : Outport  Port=5
  Act_Axis6 [deg] : Outport  Port=6
  New Data Flag (93) : Outport  Port=7
  wires:
  GT-RT CAN RX1/2 -> Demux/1
  Demux/1 -> Convert 4*uni8 to int/1(byte0)
  Demux/2 -> Convert 4*uni8 to int/2(byte1)
  Demux/3 -> Convert 4*uni8 to int/3(byte2)
  Demux/4 -> Convert 4*uni8 to int/4(byte3)
  Convert 4*uni8 to int/1(int) -> Gain/1
  Gain/1 -> Act_Axis1 [deg]/1
  Convert 4*uni8 to int1/1(int) -> Gain2/1
  Gain2/1 -> Act_Axis2  [deg]/1
  Demux/5 -> Convert 4*uni8 to int1/1(byte0)
  Demux/6 -> Convert 4*uni8 to int1/2(byte1)
  Demux/7 -> Convert 4*uni8 to int1/3(byte2)
  Demux/8 -> Convert 4*uni8 to int1/4(byte3)
  GT-RT CAN RX2/2 -> Demux1/1
  Demux1/1 -> Convert 4*uni8 to int2/1(byte0)
  Demux1/2 -> Convert 4*uni8 to int2/2(byte1)
  Demux1/3 -> Convert 4*uni8 to int2/3(byte2)
  Demux1/4 -> Convert 4*uni8 to int2/4(byte3)
  Convert 4*uni8 to int2/1(int) -> Gain6/1
  Demux1/5 -> Convert 4*uni8 to int3/1(byte0)
  Demux1/6 -> Convert 4*uni8 to int3/2(byte1)
  Demux1/7 -> Convert 4*uni8 to int3/3(byte2)
  Demux1/8 -> Convert 4*uni8 to int3/4(byte3)
  GT-RT CAN RX3/2 -> Demux2/1
  Demux2/1 -> Convert 4*uni8 to int4/1(byte0)
  Demux2/2 -> Convert 4*uni8 to int4/2(byte1)
  Demux2/3 -> Convert 4*uni8 to int4/3(byte2)
  Demux2/4 -> Convert 4*uni8 to int4/4(byte3)
  Convert 4*uni8 to int4/1(int) -> Gain3/1
  Convert 4*uni8 to int5/1(int) -> Gain4/1
  Demux2/5 -> Convert 4*uni8 to int5/1(byte0)
  Demux2/6 -> Convert 4*uni8 to int5/2(byte1)
  Demux2/7 -> Convert 4*uni8 to int5/3(byte2)
  Demux2/8 -> Convert 4*uni8 to int5/4(byte3)
  GT-RT CAN RX3/5 -> New Data Flag (93)/1
  GT-RT CAN RX1/1 -> Terminator1/1
  GT-RT CAN RX1/3 -> Terminator2/1
  GT-RT CAN RX1/4 -> Terminator3/1
  GT-RT CAN RX1/5 -> Terminator4/1
  GT-RT CAN RX1/6 -> Terminator5/1
  GT-RT CAN RX2/1 -> Terminator6/1
  GT-RT CAN RX2/3 -> Terminator7/1
  GT-RT CAN RX2/4 -> Terminator8/1
  GT-RT CAN RX2/5 -> Terminator9/1
  GT-RT CAN RX2/6 -> Terminator10/1
  GT-RT CAN RX3/1 -> Terminator11/1
  GT-RT CAN RX3/3 -> Terminator12/1
  GT-RT CAN RX3/4 -> Terminator13/1
  GT-RT CAN RX3/6 -> Terminator14/1
  Gain6/1 -> Act_Axis3  [deg]/1
  Convert 4*uni8 to int3/1(int) -> Gain1/1
  Gain1/1 -> Act_Axis4 [deg]/1
  Gain3/1 -> Act_Axis5 [deg]/1
  Gain4/1 -> Act_Axis6 [deg]/1

== system Sim_Forcing_003h_expe_infra_transz_lim/BEC (May 7, 2015)/CAN Send ==
  New data flag (93) : Inport  OutDataType=fixdt(1, 16)  OutScaling=2^0
  A1 [deg/4ms] : Inport  Port=2  OutDataType=fixdt(1, 16)  OutScaling=2^0
  A2 [deg/4ms] : Inport  Port=3  OutDataType=fixdt(1, 16)  OutScaling=2^0
  A3 [deg/4ms] : Inport  Port=4  OutDataType=fixdt(1, 16)  OutScaling=2^0
  A4 [deg/4ms] : Inport  Port=5  OutDataType=fixdt(1, 16)  OutScaling=2^0
  A5 [deg/4ms] : Inport  Port=6  OutDataType=fixdt(1, 16)  OutScaling=2^0
  A6 [deg/4ms] : Inport  Port=7  OutDataType=fixdt(1, 16)  OutScaling=2^0
  Gain{,1..5} (6 alike) : Gain  Gain=1e8  ParameterDataType=fixdt(1, 16)  ParameterScaling=2^0  OutDataType=fixdt(1, 16)  OutScaling=2^0
  If : If  IfExpression=u1 ~= 0  ShowElse=off
  If Action Subsystem1 : Subsystem  TreatAsAtomicUnit=on
  wires:
  If/1 -> If Action Subsystem1/Action
  New data flag (93)/1 -> If/1
  A1 [deg/4ms]/1 -> Gain/1
  A2 [deg/4ms]/1 -> Gain1/1
  A3 [deg/4ms]/1 -> Gain2/1
  A4 [deg/4ms]/1 -> Gain3/1
  A5 [deg/4ms]/1 -> Gain4/1
  A6 [deg/4ms]/1 -> Gain5/1
  Gain/1 -> If Action Subsystem1/1(In1)
  Gain1/1 -> If Action Subsystem1/2(In2)
  Gain2/1 -> If Action Subsystem1/3(In3)
  Gain3/1 -> If Action Subsystem1/4(In4)
  Gain4/1 -> If Action Subsystem1/5(In5)
  Gain5/1 -> If Action Subsystem1/6(In6)

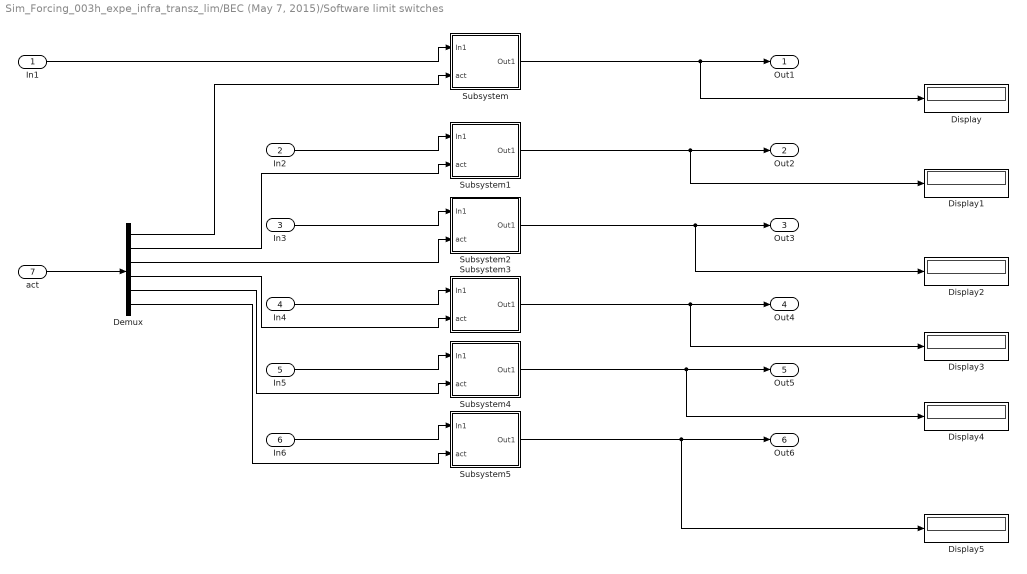
== system Sim_Forcing_003h_expe_infra_transz_lim/BEC (May 7, 2015)/Software limit switches ==
  In1 : Inport
  In2 : Inport  Port=2
  In3 : Inport  Port=3
  In4 : Inport  Port=4
  In5 : Inport  Port=5
  In6 : Inport  Port=6
  act : Inport  Port=7
  Demux : Demux  Outputs=6
  Display{,1..5} (6 alike) : Display
  Subsystem : Subsystem
  Subsystem1 : Subsystem
  Subsystem2 : Subsystem
  Subsystem3 : Subsystem
  Subsystem4 : Subsystem
  Subsystem5 : Subsystem
  Out1 : Outport
  Out2 : Outport  Port=2
  Out3 : Outport  Port=3
  Out4 : Outport  Port=4
  Out5 : Outport  Port=5
  Out6 : Outport  Port=6
  wires:
  In6/1 -> Subsystem5/1(In1)
  Subsystem5/1(Out1) -> Display5/1, Out6/1
  In5/1 -> Subsystem4/1(In1)
  Subsystem4/1(Out1) -> Display4/1, Out5/1
  In4/1 -> Subsystem3/1(In1)
  Subsystem3/1(Out1) -> Display3/1, Out4/1
  In3/1 -> Subsystem2/1(In1)
  Subsystem2/1(Out1) -> Display2/1, Out3/1
  In2/1 -> Subsystem1/1(In1)
  Subsystem1/1(Out1) -> Display1/1, Out2/1
  In1/1 -> Subsystem/1(In1)
  Subsystem/1(Out1) -> Display/1, Out1/1
  act/1 -> Demux/1
  Demux/1 -> Subsystem/2(act)
  Demux/2 -> Subsystem1/2(act)
  Demux/3 -> Subsystem2/2(act)
  Demux/4 -> Subsystem3/2(act)
  Demux/5 -> Subsystem4/2(act)
  Demux/6 -> Subsystem5/2(act)

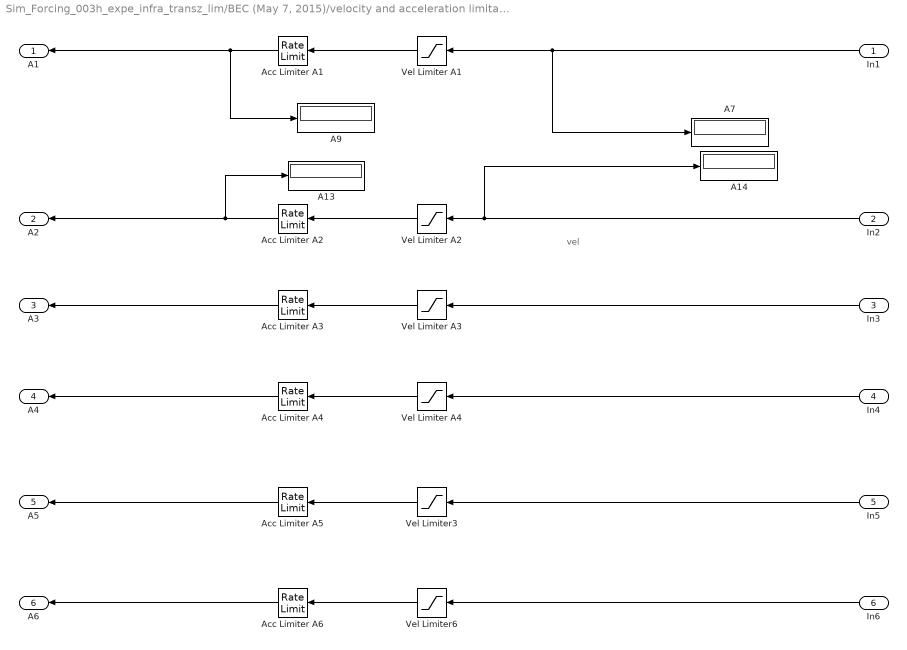
== system Sim_Forcing_003h_expe_infra_transz_lim/BEC (May 7, 2015)/velocity and acceleration limitation ==
  note: vel
  In1 : Inport
  In2 : Inport  Port=2
  In3 : Inport  Port=3
  In4 : Inport  Port=4
  In5 : Inport  Port=5
  In6 : Inport  Port=6
  A{7,9,13..14} (4 alike) : Display
  Acc Limiter A1 : RateLimiter  RisingSlewLimit=98  FallingSlewLimit=-98  SampleTimeMode=inherited
  Acc Limiter A2 : RateLimiter  RisingSlewLimit=70  FallingSlewLimit=-70  SampleTimeMode=inherited
  Acc Limiter A3 : RateLimiter  RisingSlewLimit=128  FallingSlewLimit=-128  SampleTimeMode=inherited
  Acc Limiter A4 : RateLimiter  RisingSlewLimit=33  FallingSlewLimit=-33  SampleTimeMode=inherited
  Acc Limiter A5 : RateLimiter  RisingSlewLimit=95  FallingSlewLimit=-95  SampleTimeMode=inherited
  Acc Limiter A6 : RateLimiter  RisingSlewLimit=77  FallingSlewLimit=-77  SampleTimeMode=inherited
  Vel Limiter A1 : Saturate  UpperLimit=68.34  LowerLimit=-68.34  OutDataType=fixdt(1, 16)  OutScaling=2^0
  Vel Limiter A2 : Saturate  UpperLimit=57  LowerLimit=-57  OutDataType=fixdt(1, 16)  OutScaling=2^0
  Vel Limiter A3 : Saturate  UpperLimit=69  LowerLimit=-69  OutDataType=fixdt(1, 16)  OutScaling=2^0
  Vel Limiter A4 : Saturate  UpperLimit=76  LowerLimit=-76  OutDataType=fixdt(1, 16)  OutScaling=2^0
  Vel Limiter3 : Saturate  UpperLimit=76  LowerLimit=-76  OutDataType=fixdt(1, 16)  OutScaling=2^0
  Vel Limiter6 : Saturate  UpperLimit=120  LowerLimit=-120  OutDataType=fixdt(1, 16)  OutScaling=2^0
  A1 : Outport
  A2 : Outport  Port=2
  A3 : Outport  Port=3
  A4 : Outport  Port=4
  A5 : Outport  Port=5
  A6 : Outport  Port=6
  wires:
  Acc Limiter A2/1 -> A13/1, A2/1
  Vel Limiter A2/1 -> Acc Limiter A2/1
  Acc Limiter A4/1 -> A4/1
  Vel Limiter A4/1 -> Acc Limiter A4/1
  Vel Limiter A1/1 -> Acc Limiter A1/1
  Acc Limiter A5/1 -> A5/1
  Acc Limiter A1/1 -> A9/1, A1/1
  In2/1 -> Vel Limiter A2/1, A14/1
  Vel Limiter3/1 -> Acc Limiter A5/1
  Vel Limiter A3/1 -> Acc Limiter A3/1
  Acc Limiter A3/1 -> A3/1
  Acc Limiter A6/1 -> A6/1
  In6/1 -> Vel Limiter6/1
  Vel Limiter6/1 -> Acc Limiter A6/1
  In3/1 -> Vel Limiter A3/1
  In4/1 -> Vel Limiter A4/1
  In5/1 -> Vel Limiter3/1
  In1/1 -> Vel Limiter A1/1, A7/1

== system Sim_Forcing_003h_expe_infra_transz_lim/Breaking_Control 20/07/15/Ellipse motion ==
  In1 : Inport  OutDataType=fixdt(1, 16)  OutScaling=2^0
  Constant : Constant  Value=0  OutDataType=fixdt(1, 16)  OutScaling=2^0
  Constant1 : Constant  Value=90  OutDataType=fixdt(1, 16)  OutScaling=2^0
  Constant2 : Constant  Value=30  OutDataType=fixdt(1, 16)  OutScaling=2^0
  Constant3 : Constant  Value=60  OutDataType=fixdt(1, 16)  OutScaling=2^0
  Constant4 : Constant  Value=0  OutDataType=fixdt(1, 16)  OutScaling=2^0
  Display : Display
  Display1 : Display
  Display2 : Display
  Gain : Gain  Gain=0  ParameterDataType=fixdt(1, 16)  ParameterScaling=2^0  OutDataType=fixdt(1, 16)  OutScaling=2^0
  Gain1 : Gain  ParameterDataType=fixdt(1, 16)  ParameterScaling=2^0  OutDataType=fixdt(1, 16)  OutScaling=2^0
  Gain2 : Gain  ParameterDataType=fixdt(1, 16)  ParameterScaling=2^0  OutDataType=fixdt(1, 16)  OutScaling=2^0
  Mux : Mux  Inputs=3
  Phase Shifted Sine 17th 1 : Subsystem
  Phase Shifted Sine 17th 2 : Subsystem
  Phase Shifted Sine 17th 2015 : Subsystem
  roll : Outport
  pitch : Outport  Port=2
  yaw : Outport  Port=3
  noise_rpy : Outport  Port=4
  wires:
  Phase Shifted Sine 17th 2015/1(Out sine) -> Gain/1
  Constant/1 -> Phase Shifted Sine 17th 2015/4(Phase Lag (deg))
  Constant1/1 -> Phase Shifted Sine 17th 1/4(Phase Lag (deg))
  Constant2/1 -> Phase Shifted Sine 17th 2015/2(T start), Phase Shifted Sine 17th 1/2(T start), Phase Shifted Sine 17th 2/2(T start)
  Constant3/1 -> Phase Shifted Sine 17th 2015/3(T_sin), Phase Shifted Sine 17th 1/3(T_sin), Phase Shifted Sine 17th 2/3(T_sin)
  Phase Shifted Sine 17th 1/1(Out sine) -> Gain1/1
  Gain/1 -> roll/1, Display/1, Mux/1
  Gain1/1 -> pitch/1, Display1/1, Mux/2
  In1/1 -> Phase Shifted Sine 17th 2015/1(Activate), Phase Shifted Sine 17th 1/1(Activate), Phase Shifted Sine 17th 2/1(Activate)
  Constant4/1 -> Phase Shifted Sine 17th 2/4(Phase Lag (deg))
  Gain2/1 -> yaw/1, Display2/1, Mux/3
  Phase Shifted Sine 17th 2/1(Out sine) -> Gain2/1
  Mux/1 -> noise_rpy/1

== system Sim_Forcing_003h_expe_infra_transz_lim/Breaking_Control 20/07/15/Move UP1 ==
  note: Amp X=80cm
      | Amp Z=101.26cm
      | Amp Theta=1.3deg
      | Tsin = 12s
  note: Max Amp X=75 cm
      | Max Amp Y=130 cm
  note: Max Amp Z= not77cm
      | because of overshoot
  PSI_SET : Inport
  Move UP : Inport  Port=2
  Select Set : Inport  Port=3
  dx : Inport  Port=4
  Enable : EnablePort
  Constant1 : Constant  Value=0  OutDataType=fixdt(1, 16)  OutScaling=2^0
  Constant2 : Constant  Value=50  OutDataType=fixdt(1, 16)  OutScaling=2^0
  Display6 : Display
  Multiport Switch : MultiPortSwitch  OutDataType=fixdt(1, 16)  OutScaling=2^0
  "Smooth Displacement Second-Order Filter, zeta 0.8" : Subsystem
  Switch : Switch  Criteria=u2 ~= 0  OutDataType=fixdt(1, 16)  OutScaling=2^0
  add x_offset : Subsystem
  curve : Stateflow chart
  set for optimizing pure z : Constant  Value="[258.3 -273.22;  251.45 -281.21; 244.6 -289.2]"  OutDataType=fixdt(1, 16)  OutScaling=2^0
  set for optimizing x and y : Constant  Value="[258.3 -273.22;  220 -330; 141.15 -390]"  OutDataType=fixdt(1, 16)  OutScaling=2^0
  set for optimizing z : Constant  Value="[258.3 -273.22;  240.025 -296.285; 221.75 -319.35]"  OutDataType=fixdt(1, 16)  OutScaling=2^0
  x : Outport
  z : Outport  Port=2
  psi : Outport  Port=3
  wires:
  Constant2/1 -> "Smooth Displacement Second-Order Filter, zeta 0.8"/2(T)
  PSI_SET/1 -> curve/2(psi_set)
  curve/2(z) -> z/1
  curve/3(psi) -> psi/1
  Move UP/1 -> "Smooth Displacement Second-Order Filter, zeta 0.8"/1(Step IN Reset on  either), Switch/2
  set for optimizing z/1 -> Multiport Switch/2
  set for optimizing pure z/1 -> Multiport Switch/3
  Select Set/1 -> Multiport Switch/1
  set for optimizing x and y/1 -> Multiport Switch/4
  curve/1(x) -> x/1
  Multiport Switch/1 -> add x_offset/2(set_in)
  add x_offset/1(set_out) -> curve/1(set)
  dx/1 -> add x_offset/1(x_offset), Display6/1
  "Smooth Displacement Second-Order Filter, zeta 0.8"/1(Out) -> Switch/1, curve/3(fraction)
  Constant1/1 -> Switch/3

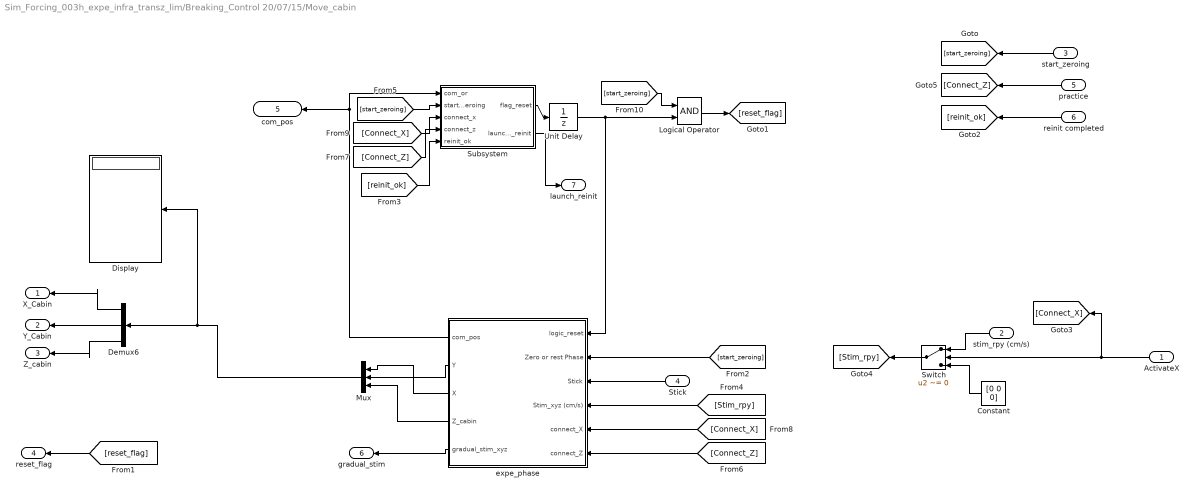
== system Sim_Forcing_003h_expe_infra_transz_lim/Breaking_Control 20/07/15/Move_cabin ==
  ActivateX : Inport
  stim_rpy (cm/s) : Inport  Port=2
  start_zeroing : Inport  Port=3
  Stick : Inport  Port=4
  practice : Inport  Port=5
  reinit completed : Inport  Port=6
  Constant : Constant  Value=[0 0 0]  OutDataType=fixdt(1, 16)  OutScaling=2^0
  Demux6 : Demux  Outputs=3
  Display : Display
  Logical Operator : Logic  AllPortsSameDT=off  OutDataTypeMode=boolean  LogicDataType=fixdt(0, 8)  OutDataTypeStr=boolean
  Mux : Mux  Inputs=3
  Subsystem : Subsystem
  Switch : Switch  Criteria=u2 ~= 0  OutDataType=fixdt(1, 16)  OutScaling=2^0
  Unit Delay : UnitDelay  SampleTime=-1
  expe_phase : Subsystem
  X_Cabin : Outport
  Y_Cabin : Outport  Port=2
  Z_cabin : Outport  Port=3
  reset_flag : Outport  Port=4
  com_pos : Outport  Port=5
  gradual_stim : Outport  Port=6
  launch_reinit : Outport  Port=7
  wires:
  Mux/1 -> Demux6/1, Display/1
  start_zeroing/1 -> [start_zeroing]
  Demux6/3 -> Z_cabin/1
  Stick/1 -> expe_phase/3(Stick)
  Subsystem/1(flag_reset) -> Unit Delay/1
  Unit Delay/1 -> expe_phase/1(logic_reset), Logical Operator/2
  [start_zeroing] -> Subsystem/2(start_zeroing)
  ActivateX/1 -> [Connect_X], Switch/2
  [Connect_X] -> Subsystem/3(connect_x)
  expe_phase/1(com_pos) -> Subsystem/1(com_or), com_pos/1
  [Connect_X] -> expe_phase/5(connect_X)
  [reset_flag] -> reset_flag/1
  [start_zeroing] -> expe_phase/2(Zero or rest Phase)
  practice/1 -> [Connect_Z]
  Switch/1 -> [Stim_rpy]
  [Stim_rpy] -> expe_phase/4(Stim_xyz (cm/s))
  [Connect_Z] -> expe_phase/6(connect_Z)
  [Connect_Z] -> Subsystem/4(connect_z)
  [start_zeroing] -> Logical Operator/1
  Logical Operator/1 -> [reset_flag]
  stim_rpy (cm/s)/1 -> Switch/1
  Constant/1 -> Switch/3
  expe_phase/5(gradual_stim_xyz) -> gradual_stim/1
  expe_phase/4(Z_cabin) -> Mux/3
  expe_phase/3(X) -> Mux/1
  expe_phase/2(Y) -> Mux/2
  Demux6/2 -> Y_Cabin/1
  Demux6/1 -> X_Cabin/1
  reinit completed/1 -> [reinit_ok]
  [reinit_ok] -> Subsystem/5(reinit_ok)
  Subsystem/2(launch_reinit) -> launch_reinit/1

== system Sim_Forcing_003h_expe_infra_transz_lim/Breaking_Control 20/07/15/Save_data1 ==
  note: we take delay_in + delay_out. We assume it remains cst
  count : Inport  OutDataType=fixdt(1, 16)  OutScaling=2^0
  delay : Inport  Port=2  OutDataType=fixdt(1, 16)  OutScaling=2^0
  Actual_pos : Inport  Port=3  OutDataType=fixdt(1, 16)  OutScaling=2^0
  com_pos : Inport  Port=4  OutDataType=fixdt(1, 16)  OutScaling=2^0
  target_velocity : Inport  Port=5  OutDataType=fixdt(1, 16)  OutScaling=2^0
  time : Inport  Port=6  OutDataType=fixdt(1, 16)  OutScaling=2^0
  IsinRestPhase : Inport  Port=7  OutDataType=fixdt(1, 16)  OutScaling=2^0
  vis_cond : Inport  Port=8  OutDataType=fixdt(1, 16)  OutScaling=2^0
  Taact : Inport  Port=9  OutDataType=fixdt(1, 16)  OutScaling=2^0
  stick before dead_zone : Inport  Port=10  OutDataType=fixdt(1, 16)  OutScaling=2^0
  gradual_stim : Inport  Port=11  OutDataType=fixdt(1, 16)  OutScaling=2^0
  noise_xyz : Inport  Port=12  OutDataType=fixdt(1, 16)  OutScaling=2^0
  Enable : EnablePort  ShowOutputPort=on
  6_DOF Visual Cab 12/06/15 : Subsystem
  Gain : Gain  ParameterDataType=fixdt(1, 16)  ParameterScaling=2^0  OutDataType=fixdt(1, 16)  OutScaling=2^0
  wires:
  delay/1 -> Gain/1
  com_pos/1 -> 6_DOF Visual Cab 12/06/15/2(Com_pos)
  count/1 -> [Cnt]
  time/1 -> [time]
  [time] -> 6_DOF Visual Cab 12/06/15/1(time)
  [targ_velocity] -> 6_DOF Visual Cab 12/06/15/5(targ_velocity)
  Gain/1 -> 6_DOF Visual Cab 12/06/15/6(delay)
  [reset] -> 6_DOF Visual Cab 12/06/15/8(reset)
  IsinRestPhase/1 -> [RestPhase]
  [RestPhase] -> 6_DOF Visual Cab 12/06/15/7(IsinRestPhase2)
  [Cnt] -> 6_DOF Visual Cab 12/06/15/4(cnt)
  vis_cond/1 -> 6_DOF Visual Cab 12/06/15/3(Vis_cond)
  target_velocity/1 -> [targ_velocity]
  Actual_pos/1 -> 6_DOF Visual Cab 12/06/15/9(act_pos)
  Taact/1 -> 6_DOF Visual Cab 12/06/15/10(Taact)
  stick before dead_zone/1 -> 6_DOF Visual Cab 12/06/15/11(Stick_before_deadzone)
  gradual_stim/1 -> 6_DOF Visual Cab 12/06/15/12(gradual_stim)
  noise_xyz/1 -> 6_DOF Visual Cab 12/06/15/13(noise_xyz)

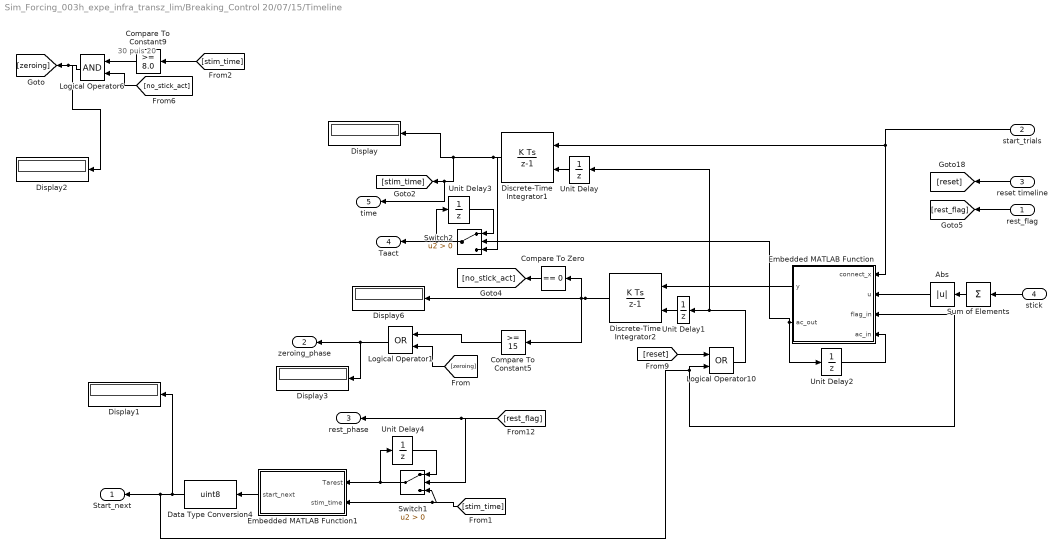
== system Sim_Forcing_003h_expe_infra_transz_lim/Breaking_Control 20/07/15/Timeline ==
  note: 30 puis 20
  rest_flag : Inport  PortDimensions=1
  start_trials : Inport  Port=2  PortDimensions=1
  reset timeline : Inport  Port=3  PortDimensions=1
  stick : Inport  Port=4
  Abs : Abs  OutDataType=fixdt(1, 16)  OutScaling=2^0
  Compare To Constant5 : simulink/Logic and Bit Operations/Compare To Constant  SystemSampleTime=-1  relop=>=  const=15  LogicOutDataTypeMode=uint8
  Compare To Constant9 : simulink/Logic and Bit Operations/Compare To Constant  SystemSampleTime=-1  relop=>=  const=8.0  LogicOutDataTypeMode=uint8
  Compare To Zero : simulink/Logic and Bit Operations/Compare To Zero  SystemSampleTime=-1  relop===  LogicOutDataTypeMode=uint8
  Data Type Conversion4 : DataTypeConversion  OutDataTypeMode=uint8  OutDataType=fixdt(1, 16)  OutScaling=2^0  OutDataTypeStr=uint8
  Discrete-Time Integrator1 : DiscreteIntegrator  ExternalReset=rising  SampleTime=0.004  LowerSaturationLimit=0  ICPrevOutput=DiscIntNeverNeededParam  ICPrevScaledInput=DiscIntNeverNeededParam
  Discrete-Time Integrator2 : DiscreteIntegrator  ExternalReset=rising  SampleTime=0.004  UpperSaturationLimit=40  LowerSaturationLimit=0  ICPrevOutput=DiscIntNeverNeededParam  ICPrevScaledInput=DiscIntNeverNeededParam
  Display{,1..3,6} (5 alike) : Display
  Embedded MATLAB Function : Stateflow chart
  Embedded MATLAB Function1 : Stateflow chart
  Logical Operator1 : Logic  Operator=OR  AllPortsSameDT=off  OutDataTypeMode=boolean  LogicDataType=fixdt(0, 8)  OutDataTypeStr=boolean
  Logical Operator10 : Logic  Operator=OR  AllPortsSameDT=off  OutDataTypeMode=boolean  LogicDataType=fixdt(0, 8)  OutDataTypeStr=boolean
  Logical Operator6 : Logic  AllPortsSameDT=off  OutDataTypeMode=boolean  LogicDataType=fixdt(0, 8)  OutDataTypeStr=boolean
  Sum of Elements : Sum  Inputs=+  OutDataType=fixdt(1, 16)  OutScaling=2^-10
  Switch1 : Switch  Criteria=u2 > Threshold  OutDataType=fixdt(1, 16)  OutScaling=2^0
  Switch2 : Switch  Criteria=u2 > Threshold  OutDataType=fixdt(1, 16)  OutScaling=2^0
  Unit Delay{,1..4} (5 alike) : UnitDelay  SampleTime=-1
  Start_next : Outport  OutDataType=fixdt(1, 16)  OutScaling=2^0
  zeroing_phase : Outport  Port=2  OutDataType=fixdt(1, 16)  OutScaling=2^0
  rest_phase : Outport  Port=3  OutDataType=fixdt(1, 16)  OutScaling=2^0
  Taact : Outport  Port=4  OutDataType=fixdt(1, 16)  OutScaling=2^0
  time : Outport  Port=5  OutDataType=fixdt(1, 16)  OutScaling=2^0
  wires:
  Discrete-Time Integrator1/1 -> Display/1, [stim_time], time/1, Switch2/3
  Embedded MATLAB Function/1(y) -> Discrete-Time Integrator2/1
  Discrete-Time Integrator2/1 -> Display6/1, Compare To Zero/1, Compare To Constant5/1
  start_trials/1 -> Embedded MATLAB Function/1(connect_x), Discrete-Time Integrator1/1
  stick/1 -> Sum of Elements/1
  Unit Delay/1 -> Discrete-Time Integrator1/2
  Unit Delay1/1 -> Discrete-Time Integrator2/2
  Sum of Elements/1 -> Abs/1
  Abs/1 -> Embedded MATLAB Function/2(u)
  Embedded MATLAB Function/2(ac_out) -> Unit Delay2/1, Switch2/2
  Unit Delay2/1 -> Embedded MATLAB Function/4(ac_in)
  Logical Operator6/1 -> [zeroing], Display2/1
  [stim_time] -> Compare To Constant9/1
  Compare To Zero/1 -> [no_stick_act]
  reset timeline/1 -> [reset]
  rest_flag/1 -> [rest_flag]
  Switch2/1 -> Taact/1, Unit Delay3/1
  Unit Delay3/1 -> Switch2/1
  [reset] -> Logical Operator10/1
  Logical Operator10/1 -> Unit Delay1/1, Unit Delay/1
  Logical Operator1/1 -> zeroing_phase/1, Display3/1
  Compare To Constant5/1 -> Logical Operator1/1
  [zeroing] -> Logical Operator1/2
  Compare To Constant9/1 -> Logical Operator6/1
  [no_stick_act] -> Logical Operator6/2
  [rest_flag] -> rest_phase/1, Switch1/2
  Embedded MATLAB Function1/1(start_next) -> Data Type Conversion4/1
  Switch1/1 -> Unit Delay4/1, Embedded MATLAB Function1/1(Tarest)
  Unit Delay4/1 -> Switch1/1
  [stim_time] -> Embedded MATLAB Function1/2(stim_time), Switch1/3
  Data Type Conversion4/1 -> Display1/1, Logical Operator10/2, Embedded MATLAB Function/3(flag_in), Start_next/1
